simulink model "My_Linear"  (R2021b)
settings: Solver=VariableStepAuto  StartTime=0.0  StopTime=simTime  RelTol=1e-3
undefined symbols (not defined in the file): Aa, Bb, Cc, Dd, RPM, TakeStep, x0
settings Model: Creator=tanzc  LastModifiedBy=tanzc

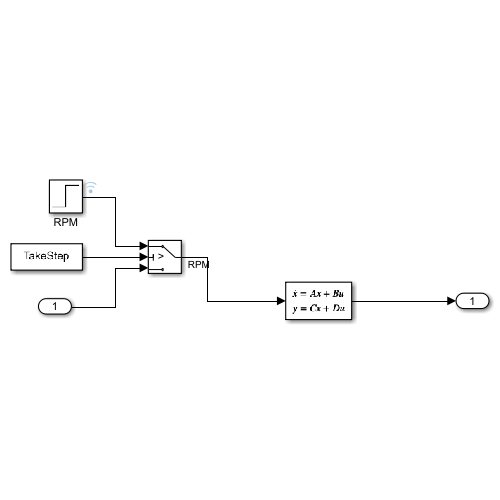
[thumbnail: Simulink's stored preview of the top-level diagram]
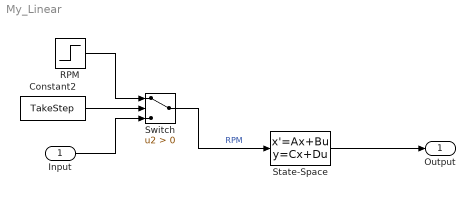
== system My_Linear ==
  Input : Inport
  Constant2 : Constant  Value=TakeStep
  RPM : Step  Time=0  After=RPM  SampleTime=0
  State-Space : StateSpace  A=Aa  B=Bb  C=Cc  D=Dd  InitialCondition=x0
  Switch : Switch  Criteria=u2 > Threshold
  Output : Outport
  wires:
  RPM/1 -> Switch/1
  Switch/1 -> State-Space/1  "RPM"
  State-Space/1 -> Output/1
  Constant2/1 -> Switch/2
  Input/1 -> Switch/3
